simulink model "test"  (R2018b)
settings: Solver=VariableStepAuto  StartTime=0.0  StopTime=10.0  RelTol=1e-3
settings Model: Creator=Bondi  LastModifiedBy=Bondi

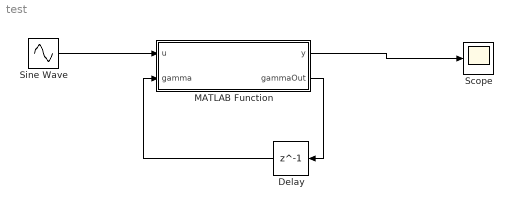
== system test ==
  Delay : Delay  DelayLength=1  InitialCondition=[0 0 0;0.2 0.2 0;0.4 0.2 0;0.4 0.4 0;0.6 0.2 0;0.6 0.4 0;0.6 0.6 0;0.8 0.2 0;0.8 0.4 0;0.8 0.6 0;0.8 0.8 0;1 0.2 0;1 0.4 0;1 0.6 0;1 0.8 0;1 1 0;1.2 0.2 0;1.2 0.4 0;1.2 0.6 0;1.2 0.8 0;1.2 1 0;1.2 1.2 0;1.4 0.2 0;1.4 0.4 0;1.4 0.6 0;1.4 0.8 0;1.4 1 0;1.4 1.2 0;1.4 1.4 0;1.6 0.2 0;1.6 0.4 0;1.6 0.6 0;1.6 0.8 0;1.6 1 0;1.6 1.2 0;1.6 1.4 0;1.6 1.6 0;1.8 0.2 0;1.8 0.4 0;1.8 0.6 0;1.8 0.8 0;1.8 1 0;1.8 1.2 0;1.8 1.4 0;1.8 1.6 0;1.8 1.8 0;2 0.2 0;2 0.4 0;2 0.6 0;2 0.8 0;2 1 0;2 1.2 0;2 1.4 0;2 1.6 0;2 1.8 0;2 2 0;2.2 0.2 0;2.2 0.4 0;2.2 0.6 0;2.2 0.8 0;2.2 1 0;2.2 1.2 0;2.2 1.4 0;2.2 1.6 0;2.2 1.8 0;2.2 2 0;2.2 2.2 0;2.4 0.2 0;2.4 0.4 0;2.4 0.6 0;2.4 0.8 0;2.4 1 0;2.4 1.2 0;2.4 1.4 0;2.4 1.6 0;2.4 1.8 0;2.4 2 0;2.4 2.2 0;2.4 2.4 0;2.6 0.2 0;2.6 0.4 0;2.6 0.6 0;2.6 0.8 0;2.6 1 0;2.6 1.2 0;2.6 1.4 0;2.6 1.6 0;2.6 1.8 0;2.6 2 0;2.6 2.2 0;2.6 2.4 0;2.6 2.6 0;2.8 0.2 0;2.8 0.4 0;2.8 0.6 0;2.8 0.8 0;2.8 1 0;2.8 1.2 0;2.8 1.4 0;2.8 1.6 0;2.8 1.8 0;2.8 2 0;2.8 2.2 0;2.8 2.4 0;2.8 2.6 0;2.8 2.8 0;3 0.2 0;3 0.4 0;3 0.6 0;3 0.8 0;3 1 0;3 1.2 0;3 1.4 0;3 1.6 0;3 1.8 0;3 2 0;3 2.2 0;3 2.4 0;3 2.6 0;3 2.8 0;3 3 0;3.2 0.2 0;3.2 0.4 0;3.2 0.6 0;3.2 0.8 0;3.2 1 0;3.2 1.2 0;3.2 1.4 0;3.2 1.6 0;3.2 1.8 0;3.2 2 0;3.2 2.2 0;3.2 2.4 0;3.2 2.6 0;3.2 2.8 0;3.2 3 0;3.2 3.2 0;3.4 0.2 0;3.4 0.4 0;3.4 0.6 0;3.4 0.8 0;3.4 1 0;3.4 1.2 0;3.4 1.4 0;3.4 1.6 0;3.4 1.8 0;3.4 2 0;3.4 2.2 0;3.4 2.4 0;3.4 2.6 0;3.4 2.8 0;3.4 3 0;3.4 3.2 0;3.4 3.4 0;3.6 0.2 0;3.6 0.4 0;3.6 0.6 0;3.6 0.8 0;3.6 1 0;3.6 1.2 0;3.6 1.4 0;3.6 1.6 0;3.6 1.8 0;3.6 2 0;3.6 2.2 0;3.6 2.4 0;3.6 2.6 0;3.6 2.8 0;3.6 3 0;3.6 3.2 0;3.6 3.4 0;3.6 3.6 0;3.8 0.2 0;3.8 0.4 0;3.8 0.6 0;3.8 0.8 0;3.8 1 0;3.8 1.2 0;3.8 1.4 0;3.8 1.6 0;3.8 1.8 0;3.8 2 0;3.8 2.2 0;3.8 2.4 0;3.8 2.6 0;3.8 2.8 0;3.8 3 0;3.8 3.2 0;3.8 3.4 0;3.8 3.6 0;3.8 3.8 0;4 0.2 0;4 0.4 0;4 0.6 0;4 0.8 0;4 1 0;4 1.2 0;4 1.4 0;4 1.6 0;4 1.8 0;4 2 0;4 2.2 0;4 2.4 0;4 2.6 0;4 2.8 0;4 3 0;4 3.2 0;4 3.4 0;4 3.6 0;4 3.8 0;4 4 0;4.2 0.2 0;4.2 0.4 0;4.2 0.6 0;4.2 0.8 0;4.2 1 0;4.2 1.2 0;4.2 1.4 0;4.2 1.6 0;4.2 1.8 0;4.2 2 0;4.2 2.2 0;4.2 2.4 0;4.2 2.6 0;4.2 2.8 0;4.2 3 0;4.2 3.2 0;4.2 3.4 0;4.2 3.6 0;4.2 3.8 0;4.2 4 0;4.2 4.2 0;4.4 0.2 0;4.4 0.4 0;4.4 0.6 0;4.4 0.8 0;4.4 1 0;4.4 1.2 0;4.4 1.4 0;4.4 1.6 0;4.4 1.8 0;4.4 2 0;4.4 2.2 0;4.4 2.4 0;4.4 2.6 0;4.4 2.8 0;4.4 3 0;4.4 3.2 0;4.4 3.4 0;4.4 3.6 0;4.4 3.8 0;4.4 4 0;4.4 4.2 0;4.4 4.4 0;4.6 0.2 0;4.6 0.4 0;4.6 0.6 0;4.6 0.8 0;4.6 1 0;4.6 1.2 0;4.6 1.4 0;4.6 1.6 0;4.6 1.8 0;4.6 2 0;4.6 2.2 0;4.6 2.4 0;4.6 2.6 0;4.6 2.8 0;4.6 3 0;4.6 3.2 0;4.6 3.4 0;4.6 3.6 0;4.6 3.8 0;4.6 4 0;4.6 4.2 0;4.6 4.4 0;4.6 4.6 0;4.8 0.2 0;4.8 0.4 0;4.8 0.6 0;4.8 0.8 0;4.8 1 0;4.8 1.2 0;4.8 1.4 0;4.8 1.6 0;4.8 1.8 0;4.8 2 0;4.8 2.2 0;4.8 2.4 0;4.8 2.6 0;4.8 2.8 0;4.8 3 0;4.8 3.2 0;4.8 3.4 0;4.8 3.6 0;4.8 3.8 0;4.8 4 0;4.8 4.2 0;4.8 4.4 0;4.8 4.6 0;4.8 4.8 0;5 0.2 0;5 0.4 0;5 0.6 0;5 0.8 0;5 1 0;5 1.2 0;5 1.4 0;5 1.6 0;5 1.8 0;5 2 0;5 2.2 0;5 2.4 0;5 2.6 0;5 2.8 0;5 3 0;5 3.2 0;5 3.4 0;5 3.6 0;5 3.8 0;5 4 0;5 4.2 0;5 4.4 0;5 4.6 0;5 4.8 0;5 5 0;5.2 0.2 0;5.2 0.4 0;5.2 0.6 0;5.2 0.8 0;5.2 1 0;5.2 1.2 0;5.2 1.4 0;5.2 1.6 0;5.2 1.8 0;5.2 2 0;5.2 2.2 0;5.2 2.4 0;5.2 2.6 0;5.2 2.8 0;5.2 3 0;5.2 3.2 0;5.2 3.4 0;5.2 3.6 0;5.2 3.8 0;5.2 4 0;5.2 4.2 0;5.2 4.4 0;5.2 4.6 0;5.2 4.8 0;5.2 5 0;5.2 5.2 0;5.4 0.2 0;5.4 0.4 0;5.4 0.6 0;5.4 0.8 0;5.4 1 0;5.4 1.2 0;5.4 1.4 0;5.4 1.6 0;5.4 1.8 0;5.4 2 0;5.4 2.2 0;5.4 2.4 0;5.4 2.6 0;5.4 2.8 0;5.4 3 0;5.4 3.2 0;5.4 3.4 0;5.4 3.6 0;5.4 3.8 0;5.4 4 0;5.4 4.2 0;5.4 4.4 0;5.4 4.6 0;5.4 4.8 0;5.4 5 0;5.4 5.2 0;5.4 5.4 0;5.6 0.2 0;5.6 0.4 0;5.6 0.6 0;5.6 0.8 0;5.6 1 0;5.6 1.2 0;5.6 1.4 0;5.6 1.6 0;5.6 1.8 0;5.6 2 0;5.6 2.2 0;5.6 2.4 0;5.6 2.6 0;5.6 2.8 0;5.6 3 0;5.6 3.2 0;5.6 3.4 0;5.6 3.6 0;5.6 3.8 0;5.6 4 0;5.6 4.2 0;5.6 4.4 0;5.6 4.6 0;5.6 4.8 0;5.6 5 0;5.6 5.2 0;5.6 5.4 0;5.6 5.6 0;5.8 0.2 0;5.8 0.4 0;5.8 0.6 0;5.8 0.8 0;5.8 1 0;5.8 1.2 0;5.8 1.4 0;5.8 1.6 0;5.8 1.8 0;5.8 2 0;5.8 2.2 0;5.8 2.4 0;5.8 2.6 0;5.8 2.8 0;5.8 3 0;5.8 3.2 0;5.8 3.4 0;5.8 3.6 0;5.8 3.8 0;5.8 4 0;5.8 4.2 0;5.8 4.4 0;5.8 4.6 0 ...(+7789 chars)]
  MATLAB Function : MATLAB Function  TreatAsAtomicUnit=on
  Scope : Scope
  Sine Wave : Sin  Amplitude=5  Bias=5  Frequency=2*pi  SampleTime=0
  wires:
  MATLAB Function/2(gammaOut) -> Delay/1
  Delay/1 -> MATLAB Function/2(gamma)
  Sine Wave/1 -> MATLAB Function/1(u)
  MATLAB Function/1(y) -> Scope/1

== matlab function test/MATLAB Function ==
  data: u input; y output; gamma input; gammaOut output
function [y, gammaOut] = fcn(u,gamma)

    mu = ones(length(gamma),1);
    [y,gammaOut] = preisach_v1(u,gamma,mu);
